simulink model "LaneSimulationV1"  (R2021b)
settings: Solver=VariableStepAuto  StartTime=0.0  StopTime=10.0  RelTol=1e-3
values from neighbouring files (symbols this model uses):
  Np = 10    [acc_plot_backup.m]
  s_path = [0 1.10508939428 2.2141958029 3.32141571172 4.42705301151 5.53154548532 6.63517443471 7.73808041313 8.84055018688 9.94289959674 11.0453539299 12.1480581097 ... (1001 elements, 1001x1)]    [200_100radius.mat]    (also in LV_Clothoid_S_Turn_path.mat = [0 0.966832089581 1.93621320584 2.90214024471 3.86476766313 ; NEDC_path.mat = [0 0.414605943146 0.832514087334 1.25401518562 1.68216660344; Straight_East_into_curve.mat = [0 1.65770560069 3.32192925577 4.98420060507 6.64484613518 8; acc_plot_backup.m = Station_HV_m)
  X_path = [0 1.10508939428 2.2141958029 3.32141571172 4.42705301151 5.53154548532 6.63517443471 7.73808041313 8.84055018688 9.94289959674 11.0453539299 12.1480581097 ... (1001 elements, 1001x1)]    [200_100radius.mat]    (also in LV_Clothoid_S_Turn_path.mat = [-10 -9.03316791042 -8.06378679416 -7.09785975529 -6.1352323; NEDC_path.mat = [0 0.414605943146 0.832514087334 1.25401518562 1.68216660344; Straight_East_into_curve.mat = [0 1.65770560069 3.32192925577 4.98420060507 6.64484613518 8; acc_plot_backup.m = X_HV_m)
  Y_path = [0 -1.70364610795e-18 -7.41532896709e-18 1.46822109542e-17 4.74557362791e-17 6.12980216762e-17 9.25043977736e-17 1.24088240159e-16 1.5099156923e-16 1.7058517853e-16 1.90629227614e-16 2.09673434424e-16 ... (1001 elements, 1001x1)]    [200_100radius.mat]    (also in LV_Clothoid_S_Turn_path.mat = [0 -8.46153035536e-19 5.07382551045e-18 2.07356032218e-17 3.; NEDC_path.mat = [0 -3.50680326162e-18 -2.14111304971e-18 3.38197671014e-18 3; Straight_East_into_curve.mat = [0 1.29197709199e-18 2.81882429322e-18 3.49020462564e-17 6.7; acc_plot_backup.m = Y_HV_m)
undefined symbols (not defined in the file or in its folder): AES_pre_time, speed, t_start, Ts_MPC
(part 2 of 12)

== matlab function LaneSimulationV1/ISO_Curve_road ==
  data: StationPath_m_CarSim input; LongitudinalSpeed_mps_CarSim input; LongitudinalAcceleration_mps2_CarSim input; YawAngle_rad_CarSim input; GlobalX_m_CarSim input; GlobalY_m_CarSim input; CL output size=[1 3]; CR output size=[1 3]; CC output size=[1 3]; DesiredPath_x_m output; DesiredPath_y_m output; CC0 output; CC1 output; CC2 output; CL0 output; CL1 output; CL2 output; CR0 output; CR1 output; CR2 output
function [CL,CR,CC,DesiredPath_x_m,DesiredPath_y_m,CC0,CC1,CC2,CL0,CL1,CL2,CR0,CR1,CR2] = Camera_emulator(StationPath_m_CarSim,LongitudinalSpeed_mps_CarSim,LongitudinalAcceleration_mps2_CarSim,YawAngle_rad_CarSim,GlobalX_m_CarSim,GlobalY_m_CarSim)
%% Global coordinate 
%%直線
